simulink model "Quadcopter_V6"  (R2024b)
settings: Solver=FixedStepAuto  StartTime=0.0  StopTime=72  FixedStep=0.01  RelTol=1e-3  EnableMultiTasking=on
InitFcn:
  | QC_Params
values from neighbouring files (symbols this model uses):
  A_drag = [Ax 0  0 ... (first row only)    [QC_Params.m]
  b = 1.140e-7    (= 1.14e-07)    [QC_Params.m]
  g = 9.81    [QC_Params.m]
  grav = [0; 0; g]    [QC_Params.m]
  Ixx = 4.856e-3    (= 0.004856)    [QC_Params.m]
  Iyy = 4.856e-3    (= 0.004856)    [QC_Params.m]
  Izz = 8.801e-3    (= 0.008801)    [QC_Params.m]
  k = 2.980e-6    (= 2.98e-06)    [QC_Params.m]
  l = 0.225    [QC_Params.m]
  m = 0.468    [QC_Params.m]
  Psi = 0    [QC_Params.m]
  traj_markers = zeros(N, 8)    [QC_Params.m]
libraries: slpidlib x6, sharedtransform x1, uavutilslib x1
settings Model: Creator=acer  LastModifiedBy=acer

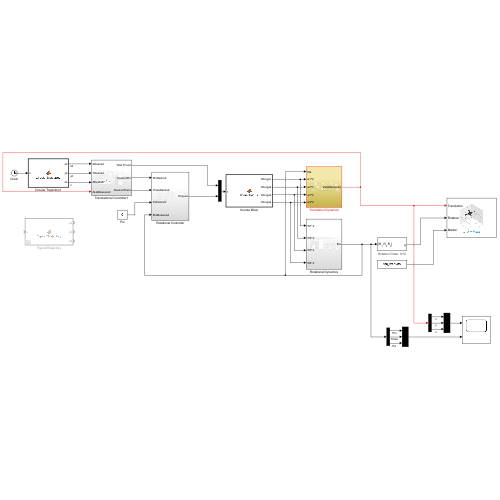
[thumbnail: Simulink's stored preview of the top-level diagram]
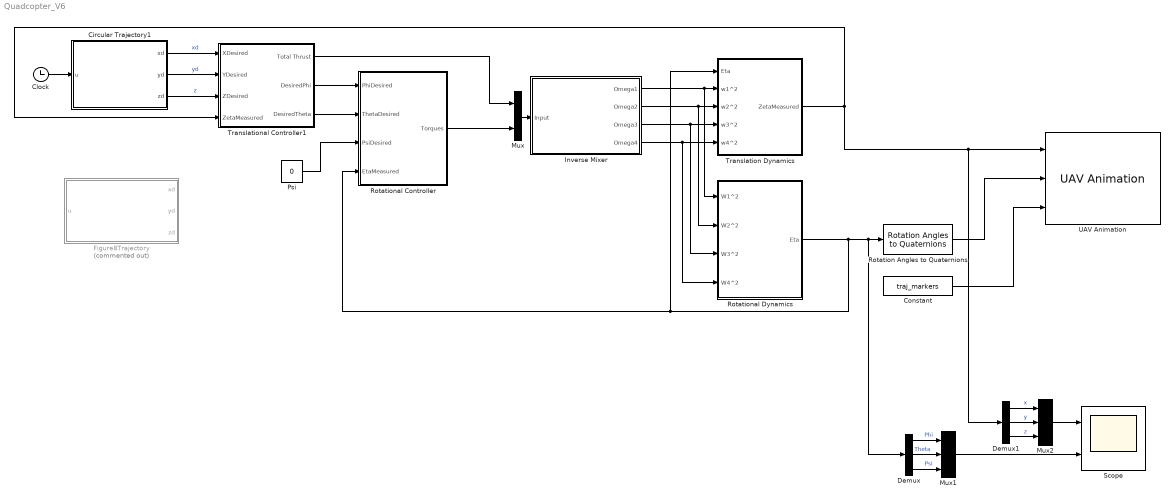
== system Quadcopter_V6 ==
  Circular Trajectory1 : MATLAB Function  TreatAsAtomicUnit=on
  Clock : Clock
  Constant : Constant  Value=traj_markers
  Demux : Demux  Outputs=3
  Demux1 : Demux  Outputs=3
  Figure8Trajectory : MATLAB Function  Commented=on  TreatAsAtomicUnit=on
  Inverse Mixer : MATLAB Function  TreatAsAtomicUnit=on
  Mux : Mux  Inputs=2
  Mux1 : Mux  Inputs=3
  Mux2 : Mux  Inputs=3
  Psi : Constant  Value=0
  Rotation Angles to Quaternions : sharedtransform/Rotation Angles to Quaternions  rotationOrder=XYZ  aMode=aMode
  Rotational Controller : Subsystem
  Rotational Dynamics : Subsystem
  Scope : Scope  NumInputPorts=2
  Translation Dynamics : Subsystem
  Translational Controller1 : Subsystem
  UAV Animation : uavutilslib/UAV Animation  NumUAV=1  DynamicUAVConfig=off  UAVType=Multirotor  UAVSize=2  UAVColor=[1 0 0]  UAVTrajectoryAlpha=1  InertialZDirection=Up  RotationFormat=Quaternion  DrawMarkers=on  SampleTime=-1
  wires:
  Inverse Mixer/1(Omega1) -> Rotational Dynamics/1(W1^2), Translation Dynamics/2(w1^2)
  Inverse Mixer/2(Omega2) -> Rotational Dynamics/2(W2^2), Translation Dynamics/3(w2^2)
  Inverse Mixer/3(Omega3) -> Rotational Dynamics/3(W3^2), Translation Dynamics/4(w3^2)
  Rotational Dynamics/1(Eta) -> Demux/1, Rotation Angles to Quaternions/1, Rotational Controller/4(EtaMeasured), Translation Dynamics/1(Eta)
  Mux/1 -> Inverse Mixer/1(Input)
  Inverse Mixer/4(Omega4) -> Rotational Dynamics/4(W4^2), Translation Dynamics/5(w4^2)
  Rotational Controller/1(Torques) -> Mux/2
  Translational Controller1/1(Total Thrust) -> Mux/1
  Translational Controller1/2(DesiredPhi) -> Rotational Controller/1(PhiDesired)
  Translational Controller1/3(DesiredTheta) -> Rotational Controller/2(ThetaDesired)
  Psi/1 -> Rotational Controller/3(PsiDesired)
  Constant/1 -> UAV Animation/3
  Circular Trajectory1/3(zd) -> Translational Controller1/3(ZDesired)  "z"
  Circular Trajectory1/1(xd) -> Translational Controller1/1(XDesired)  "xd"
  Circular Trajectory1/2(yd) -> Translational Controller1/2(YDesired)  "yd"
  Translation Dynamics/1(ZetaMeasured) -> Translational Controller1/4(ZetaMeasured), Demux1/1, UAV Animation/1
  Clock/1 -> Circular Trajectory1/1(u)
  Rotation Angles to Quaternions/1 -> UAV Animation/2
  Mux1/1 -> Scope/2
  Demux/2 -> Mux1/2  "Theta"
  Demux/1 -> Mux1/1  "Phi"
  Demux/3 -> Mux1/3  "Psi"
  Demux1/1 -> Mux2/1  "x"
  Demux1/2 -> Mux2/2  "y"
  Demux1/3 -> Mux2/3  "z"
  Mux2/1 -> Scope/1

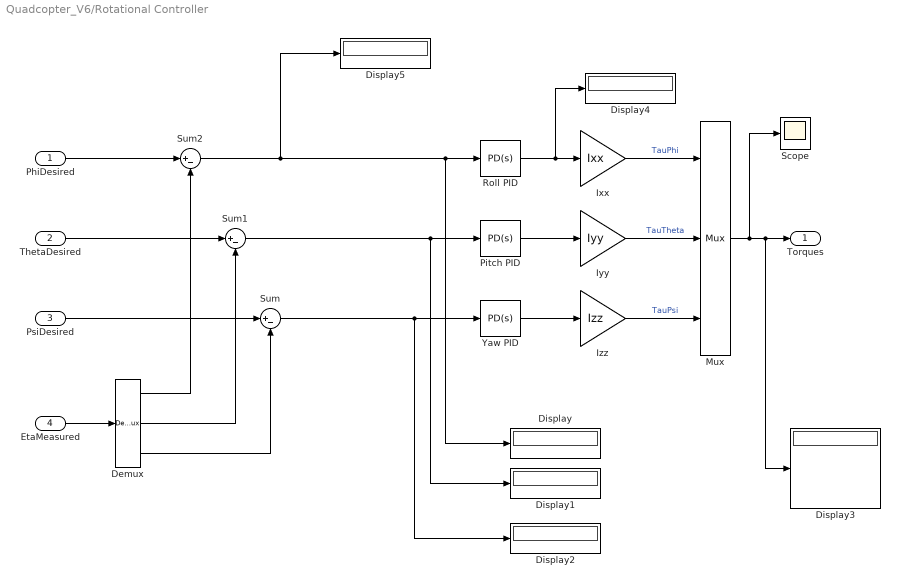
== system Quadcopter_V6/Rotational Controller ==
  PhiDesired : Inport
  ThetaDesired : Inport  Port=2
  PsiDesired : Inport  Port=3
  EtaMeasured : Inport  Port=4
  Demux : Demux  Outputs=3
  Display{,1..5} (6 alike) : Display
  Ixx : Gain  Gain=Ixx
  Iyy : Gain  Gain=Iyy
  Izz : Gain  Gain=Izz
  Mux : Mux  Inputs=3
  Pitch PID : slpidlib/PID Controller  Controller=PD  Form=Parallel  TimeDomain=Continuous-time  UseExternalTs=off  SampleTime=-1  IntegratorMethod=Forward Euler  FilterMethod=Forward Euler  ControllerParametersSource=internal  P=0.2  I=1.75  UseKiTs=off  D=10  UseExternalDerivativeSource=off  N=100  UseFilter=on  TunerSelectOption=Transfer Function Based (PID Tuner App)  InitialConditionSource=internal  InitialConditionForIntegrator=0  InitialConditionForFilter=0  DifferentiatorICPrevScaledInput=0  ExternalReset=none  TrackingMode=off  Kt=1  LimitOutput=off  SatLimitsSource=internal  UpperSaturationLimit=0.5  LowerSaturationLimit=-0.5  LinearizeAsGain=on  AntiWindupMode=none  Kb=1  LimitIntegrator=off  UpperIntegratorSaturationLimit=inf  LowerIntegratorSaturationLimit=-inf  POutMin=[]  POutMax=[]  IOutMin=[]  IOutMax=[]  DOutMin=[]  DOutMax=[]  NOutMin=[]  NOutMax=[]  SumOutMin=[]  SumOutMax=[]  SaturationOutMin=[]  SaturationOutMax=[]  PParamMin=[]  PParamMax=[]  IParamMin=[]  IParamMax=[]  DParamMin=[]  DParamMax=[]  NParamMin=[]  NParamMax=[]  KbParamMin=[]  KbParamMax=[]  KtParamMin=[]  KtParamMax=[]  KbOutMin=[]  KbOutMax=[]  KtOutMin=[]  KtOutMax=[]  IntegratorOutMin=[]  IntegratorOutMax=[]  FilterOutMin=[]  FilterOutMax=[]  SumI1OutMin=[]  SumI1OutMax=[]  SumI2OutMin=[]  SumI2OutMax=[]  SumI3OutMin=[]  SumI3OutMax=[]  SumI4OutMin=[]  SumI4OutMax=[]  SumDOutMin=[]  SumDOutMax=[]  DifferentiatorOutMin=[]  DifferentiatorOutMax=[]  FilterDiffOutCoefMin=[]  FilterDiffOutCoefMax=[]  ReciprocalOutMin=[]  ReciprocalOutMax=[]  SumDenOutMin=[]  SumDenOutMax=[]  SumNumOutMin=[]  SumNumOutMax=[]  DivideOutMin=[]  DivideOutMax=[]  UdiffTsProdOutMin=[]  UdiffTsProdOutMax=[]  NTsProdOutMin=[]  NTsProdOutMax=[]  UintegralTsProdOutMin=[]  UintegralTsProdOutMax=[]  UngainTsProdOutMin=[]  UngainTsProdOutMax=[]  ClampingZeroOutDataTypeStr=Inherit: Inherit via back propagation  ClampingZeroOutMin=[]  ClampingZeroOutMax=[]  FilterDenConstantOutDataTypeStr=Inherit: Inherit via back propagation  FilterDenConstantOutMin=[]  FilterDenConstantOutMax=[]  PCopyOutDataTypeStr=Inherit: Inherit via back propagation  PCopyOutMin=[]  PCopyOutMax=[]  NCopyOutDataTypeStr=Inherit: Inherit via back propagation  NCopyOutMin=[]  NCopyOutMax=[]  IntegratorContinuousStateAttributes=''  IntegratorStateMustResolveToSignalObject=off  IntegratorRTWStateStorageClass=Auto  FilterContinuousStateAttributes=''  FilterStateMustResolveToSignalObject=off  FilterRTWStateStorageClass=Auto  ParallelPVariant=InternalParameters  IdealPVariant=Disabled  IVariant=Disabled  DVariant=InternalParameters  IntegratorVariant=Disabled  SatVariant=Disabled  AWVariant=Disabled  PCopyVariant=Disabled  TRVariant=Disabled  FdbkBlocksVariant=Forward  IdealPFdbkVariant=Disabled  SatFdbkVariant=Disabled  DerivativeFilterVariant=ContFilter  NVariant=InternalParameters  NCopyVariant=Disabled  FilterICVariant=InternalICsFilter  IntegratorICVariant=Disabled  ExternalResetVariant=Disabled  TRSumVariant=Passthrough  SumFdbkVariant=Disabled  SumVariant=Sum_PD  TsampFilterVariant=InternalTs  TsampNgainVariant=Passthrough  TsampIntegralVariant=Disabled_SignalSpec  ExternalSaturationOutDataTypeStr=Inherit: Same as second input  DerivativeSourceVariant=ErrorSignal  PreIntVariant=InternalPreInt
  Roll PID : slpidlib/PID Controller  Controller=PD  Form=Parallel  TimeDomain=Continuous-time  UseExternalTs=off  SampleTime=-1  IntegratorMethod=Forward Euler  FilterMethod=Forward Euler  ControllerParametersSource=internal  P=0.2  I=0.15  UseKiTs=off  D=10  UseExternalDerivativeSource=off  N=100  UseFilter=on  TunerSelectOption=Transfer Function Based (PID Tuner App)  InitialConditionSource=internal  InitialConditionForIntegrator=0  InitialConditionForFilter=0  DifferentiatorICPrevScaledInput=0  ExternalReset=none  TrackingMode=off  Kt=1  LimitOutput=off  SatLimitsSource=internal  UpperSaturationLimit=0.5  LowerSaturationLimit=-0.5  LinearizeAsGain=on  AntiWindupMode=none  Kb=1  LimitIntegrator=off  UpperIntegratorSaturationLimit=inf  LowerIntegratorSaturationLimit=-inf  POutMin=[]  POutMax=[]  IOutMin=[]  IOutMax=[]  DOutMin=[]  DOutMax=[]  NOutMin=[]  NOutMax=[]  SumOutMin=[]  SumOutMax=[]  SaturationOutMin=[]  SaturationOutMax=[]  PParamMin=[]  PParamMax=[]  IParamMin=[]  IParamMax=[]  DParamMin=[]  DParamMax=[]  NParamMin=[]  NParamMax=[]  KbParamMin=[]  KbParamMax=[]  KtParamMin=[]  KtParamMax=[]  KbOutMin=[]  KbOutMax=[]  KtOutMin=[]  KtOutMax=[]  IntegratorOutMin=[]  IntegratorOutMax=[]  FilterOutMin=[]  FilterOutMax=[]  SumI1OutMin=[]  SumI1OutMax=[]  SumI2OutMin=[]  SumI2OutMax=[]  SumI3OutMin=[]  SumI3OutMax=[]  SumI4OutMin=[]  SumI4OutMax=[]  SumDOutMin=[]  SumDOutMax=[]  DifferentiatorOutMin=[]  DifferentiatorOutMax=[]  FilterDiffOutCoefMin=[]  FilterDiffOutCoefMax=[]  ReciprocalOutMin=[]  ReciprocalOutMax=[]  SumDenOutMin=[]  SumDenOutMax=[]  SumNumOutMin=[]  SumNumOutMax=[]  DivideOutMin=[]  DivideOutMax=[]  UdiffTsProdOutMin=[]  UdiffTsProdOutMax=[]  NTsProdOutMin=[]  NTsProdOutMax=[]  UintegralTsProdOutMin=[]  UintegralTsProdOutMax=[]  UngainTsProdOutMin=[]  UngainTsProdOutMax=[]  ClampingZeroOutDataTypeStr=Inherit: Inherit via back propagation  ClampingZeroOutMin=[]  ClampingZeroOutMax=[]  FilterDenConstantOutDataTypeStr=Inherit: Inherit via back propagation  FilterDenConstantOutMin=[]  FilterDenConstantOutMax=[]  PCopyOutDataTypeStr=Inherit: Inherit via back propagation  PCopyOutMin=[]  PCopyOutMax=[]  NCopyOutDataTypeStr=Inherit: Inherit via back propagation  NCopyOutMin=[]  NCopyOutMax=[]  IntegratorContinuousStateAttributes=''  IntegratorStateMustResolveToSignalObject=off  IntegratorRTWStateStorageClass=Auto  FilterContinuousStateAttributes=''  FilterStateMustResolveToSignalObject=off  FilterRTWStateStorageClass=Auto  ParallelPVariant=InternalParameters  IdealPVariant=Disabled  IVariant=Disabled  DVariant=InternalParameters  IntegratorVariant=Disabled  SatVariant=Disabled  AWVariant=Disabled  PCopyVariant=Disabled  TRVariant=Disabled  FdbkBlocksVariant=Forward  IdealPFdbkVariant=Disabled  SatFdbkVariant=Disabled  DerivativeFilterVariant=ContFilter  NVariant=InternalParameters  NCopyVariant=Disabled  FilterICVariant=InternalICsFilter  IntegratorICVariant=Disabled  ExternalResetVariant=Disabled  TRSumVariant=Passthrough  SumFdbkVariant=Disabled  SumVariant=Sum_PD  TsampFilterVariant=InternalTs  TsampNgainVariant=Passthrough  TsampIntegralVariant=Disabled_SignalSpec  ExternalSaturationOutDataTypeStr=Inherit: Same as second input  DerivativeSourceVariant=ErrorSignal  PreIntVariant=InternalPreInt
  Scope : Scope
  Sum : Sum  Inputs=|+-
  Sum1 : Sum  Inputs=|+-
  Sum2 : Sum  Inputs=|+-
  Yaw PID : slpidlib/PID Controller  Controller=PD  Form=Parallel  TimeDomain=Continuous-time  UseExternalTs=off  SampleTime=-1  IntegratorMethod=Forward Euler  FilterMethod=Forward Euler  ControllerParametersSource=internal  P=0.2  I=1  UseKiTs=off  D=10  UseExternalDerivativeSource=off  N=100  UseFilter=on  TunerSelectOption=Transfer Function Based (PID Tuner App)  InitialConditionSource=internal  InitialConditionForIntegrator=0  InitialConditionForFilter=0  DifferentiatorICPrevScaledInput=0  ExternalReset=none  TrackingMode=off  Kt=1  LimitOutput=off  SatLimitsSource=internal  UpperSaturationLimit=2*pi  LowerSaturationLimit=-2*pi  LinearizeAsGain=on  AntiWindupMode=none  Kb=1  LimitIntegrator=off  UpperIntegratorSaturationLimit=inf  LowerIntegratorSaturationLimit=-inf  POutMin=[]  POutMax=[]  IOutMin=[]  IOutMax=[]  DOutMin=[]  DOutMax=[]  NOutMin=[]  NOutMax=[]  SumOutMin=[]  SumOutMax=[]  SaturationOutMin=[]  SaturationOutMax=[]  PParamMin=[]  PParamMax=[]  IParamMin=[]  IParamMax=[]  DParamMin=[]  DParamMax=[]  NParamMin=[]  NParamMax=[]  KbParamMin=[]  KbParamMax=[]  KtParamMin=[]  KtParamMax=[]  KbOutMin=[]  KbOutMax=[]  KtOutMin=[]  KtOutMax=[]  IntegratorOutMin=[]  IntegratorOutMax=[]  FilterOutMin=[]  FilterOutMax=[]  SumI1OutMin=[]  SumI1OutMax=[]  SumI2OutMin=[]  SumI2OutMax=[]  SumI3OutMin=[]  SumI3OutMax=[]  SumI4OutMin=[]  SumI4OutMax=[]  SumDOutMin=[]  SumDOutMax=[]  DifferentiatorOutMin=[]  DifferentiatorOutMax=[]  FilterDiffOutCoefMin=[]  FilterDiffOutCoefMax=[]  ReciprocalOutMin=[]  ReciprocalOutMax=[]  SumDenOutMin=[]  SumDenOutMax=[]  SumNumOutMin=[]  SumNumOutMax=[]  DivideOutMin=[]  DivideOutMax=[]  UdiffTsProdOutMin=[]  UdiffTsProdOutMax=[]  NTsProdOutMin=[]  NTsProdOutMax=[]  UintegralTsProdOutMin=[]  UintegralTsProdOutMax=[]  UngainTsProdOutMin=[]  UngainTsProdOutMax=[]  ClampingZeroOutDataTypeStr=Inherit: Inherit via back propagation  ClampingZeroOutMin=[]  ClampingZeroOutMax=[]  FilterDenConstantOutDataTypeStr=Inherit: Inherit via back propagation  FilterDenConstantOutMin=[]  FilterDenConstantOutMax=[]  PCopyOutDataTypeStr=Inherit: Inherit via back propagation  PCopyOutMin=[]  PCopyOutMax=[]  NCopyOutDataTypeStr=Inherit: Inherit via back propagation  NCopyOutMin=[]  NCopyOutMax=[]  IntegratorContinuousStateAttributes=''  IntegratorStateMustResolveToSignalObject=off  IntegratorRTWStateStorageClass=Auto  FilterContinuousStateAttributes=''  FilterStateMustResolveToSignalObject=off  FilterRTWStateStorageClass=Auto  ParallelPVariant=InternalParameters  IdealPVariant=Disabled  IVariant=Disabled  DVariant=InternalParameters  IntegratorVariant=Disabled  SatVariant=Disabled  AWVariant=Disabled  PCopyVariant=Disabled  TRVariant=Disabled  FdbkBlocksVariant=Forward  IdealPFdbkVariant=Disabled  SatFdbkVariant=Disabled  DerivativeFilterVariant=ContFilter  NVariant=InternalParameters  NCopyVariant=Disabled  FilterICVariant=InternalICsFilter  IntegratorICVariant=Disabled  ExternalResetVariant=Disabled  TRSumVariant=Passthrough  SumFdbkVariant=Disabled  SumVariant=Sum_PD  TsampFilterVariant=InternalTs  TsampNgainVariant=Passthrough  TsampIntegralVariant=Disabled_SignalSpec  ExternalSaturationOutDataTypeStr=Inherit: Same as second input  DerivativeSourceVariant=ErrorSignal  PreIntVariant=InternalPreInt
  Torques : Outport
  wires:
  EtaMeasured/1 -> Demux/1
  PsiDesired/1 -> Sum/1
  ThetaDesired/1 -> Sum1/1
  PhiDesired/1 -> Sum2/1
  Sum2/1 -> Display5/1, Display/1, Roll PID/1
  Sum1/1 -> Display1/1, Pitch PID/1
  Sum/1 -> Display2/1, Yaw PID/1
  Roll PID/1 -> Display4/1, Ixx/1
  Pitch PID/1 -> Iyy/1
  Yaw PID/1 -> Izz/1
  Izz/1 -> Mux/3  "TauPsi"
  Iyy/1 -> Mux/2  "TauTheta"
  Ixx/1 -> Mux/1  "TauPhi"
  Mux/1 -> Scope/1, Display3/1, Torques/1
  Demux/1 -> Sum2/2
  Demux/2 -> Sum1/2
  Demux/3 -> Sum/2

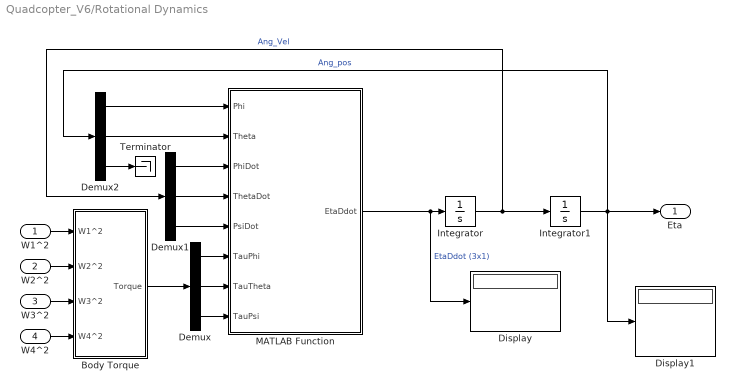
== system Quadcopter_V6/Rotational Dynamics ==
  W1^2 : Inport
  W2^2 : Inport  Port=2
  W3^2 : Inport  Port=3
  W4^2 : Inport  Port=4
  Body Torque : Subsystem
  Demux : Demux  Outputs=3
  Demux1 : Demux  Outputs=3
  Demux2 : Demux  Outputs=3
  Display : Display
  Display1 : Display
  Integrator : Integrator  InitialCondition=[0;0;0]  IgnoreLimit=on
  Integrator1 : Integrator  InitialCondition=[0;0;0]
  MATLAB Function : MATLAB Function  TreatAsAtomicUnit=on
  Terminator : Terminator
  Eta : Outport
  wires:
  W1^2/1 -> Body Torque/1(W1^2)
  W2^2/1 -> Body Torque/2(W2^2)
  W3^2/1 -> Body Torque/3(W3^2)
  W4^2/1 -> Body Torque/4(W4^2)
  Body Torque/1(Torque) -> Demux/1
  Integrator/1 -> Integrator1/1, Demux1/1  "Ang_Vel"
  Integrator1/1 -> Display1/1, Demux2/1, Eta/1  "Ang_pos"
  Demux2/1 -> MATLAB Function/1(Phi)
  Demux2/3 -> Terminator/1
  Demux/1 -> MATLAB Function/6(TauPhi)
  Demux/2 -> MATLAB Function/7(TauTheta)
  Demux/3 -> MATLAB Function/8(TauPsi)
  Demux1/2 -> MATLAB Function/4(ThetaDot)
  Demux1/1 -> MATLAB Function/3(PhiDot)
  Demux2/2 -> MATLAB Function/2(Theta)
  Demux1/3 -> MATLAB Function/5(PsiDot)
  MATLAB Function/1(EtaDdot) -> Display/1, Integrator/1  "EtaDdot (3x1)"

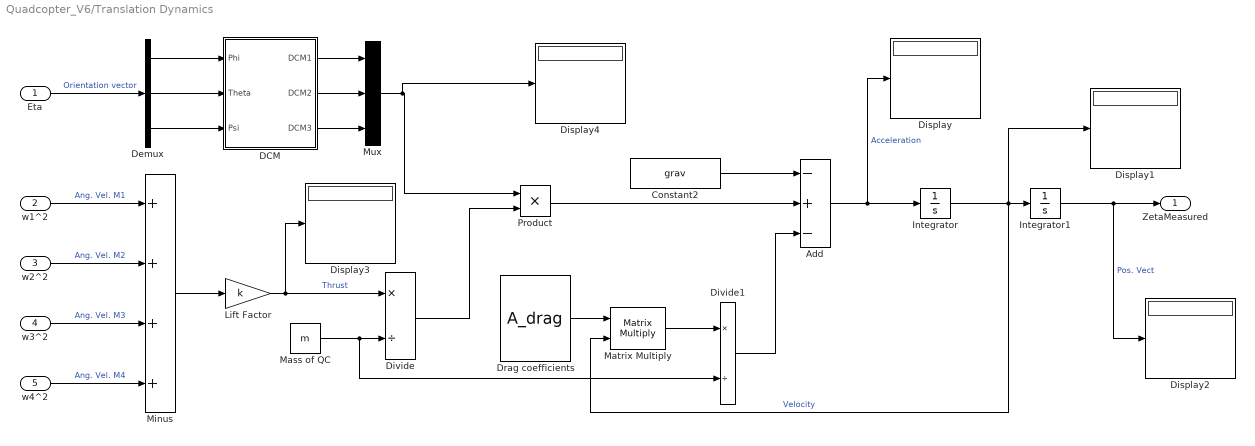
== system Quadcopter_V6/Translation Dynamics ==
  Eta : Inport
  w1^2 : Inport  Port=2
  w2^2 : Inport  Port=3
  w3^2 : Inport  Port=4
  w4^2 : Inport  Port=5
  Add : Sum  Inputs=-+-
  Constant2 : Constant  Value=grav
  "DCM " : MATLAB Function  TreatAsAtomicUnit=on
  Demux : Demux  Outputs=3
  Display{,1..4} (5 alike) : Display
  Divide : Product  Inputs=*/
  Divide1 : Product  Inputs=*/
  Drag coefficients : Constant  Value=A_drag
  Integrator : Integrator  InitialCondition=[0;0;0]
  Integrator1 : Integrator  InitialCondition=[0;0;0]
  Lift Factor : Gain  Gain=k
  Mass of QC : Constant  Value=m
  Matrix Multiply : Product  Multiplication=Matrix(*)
  Minus : Sum  Inputs=++++
  Mux : Mux  Inputs=3
  Product : Product
  ZetaMeasured : Outport
  wires:
  w1^2/1 -> Minus/1  "Ang. Vel. M1"
  w2^2/1 -> Minus/2  "Ang. Vel. M2"
  w3^2/1 -> Minus/3  "Ang. Vel. M3"
  w4^2/1 -> Minus/4  "Ang. Vel. M4"
  Minus/1 -> Lift Factor/1
  Eta/1 -> Demux/1  "Orientation vector"
  Demux/3 -> "DCM "/3(Psi)
  Demux/2 -> "DCM "/2(Theta)
  Demux/1 -> "DCM "/1(Phi)
  Lift Factor/1 -> Display3/1, Divide/1  "Thrust"
  Mass of QC/1 -> Divide1/2, Divide/2
  Divide/1 -> Product/2
  Drag coefficients/1 -> Matrix Multiply/1
  Matrix Multiply/1 -> Divide1/1
  Constant2/1 -> Add/1
  Product/1 -> Add/2
  Divide1/1 -> Add/3
  Add/1 -> Display/1, Integrator/1  "Acceleration"
  Integrator/1 -> Display1/1, Matrix Multiply/2, Integrator1/1  "Velocity"
  Integrator1/1 -> Display2/1, ZetaMeasured/1  "Pos. Vect"
  Mux/1 -> Display4/1, Product/1
  "DCM "/1(DCM1) -> Mux/1
  "DCM "/2(DCM2) -> Mux/2
  "DCM "/3(DCM3) -> Mux/3

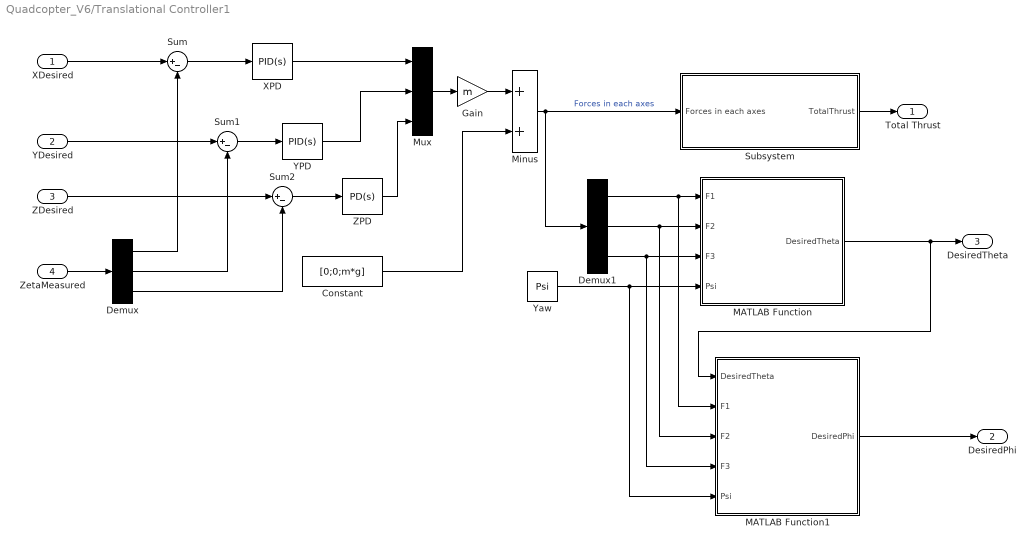
== system Quadcopter_V6/Translational Controller1 ==
  XDesired : Inport
  YDesired : Inport  Port=2
  ZDesired : Inport  Port=3
  ZetaMeasured : Inport  Port=4
  Constant : Constant  Value=[0;0;m*g]
  Demux : Demux  Outputs=3
  Demux1 : Demux  Outputs=3
  Gain : Gain  Gain=m
  MATLAB Function : MATLAB Function  TreatAsAtomicUnit=on
  MATLAB Function1 : MATLAB Function  TreatAsAtomicUnit=on
  Minus : Sum
  Mux : Mux  Inputs=3
  Subsystem : Subsystem
  Sum : Sum  Inputs=|+-
  Sum1 : Sum  Inputs=|+-
  Sum2 : Sum  Inputs=|+-
  XPD : slpidlib/PID Controller  Controller=PID  Form=Parallel  TimeDomain=Continuous-time  UseExternalTs=off  SampleTime=-1  IntegratorMethod=Forward Euler  FilterMethod=Forward Euler  ControllerParametersSource=internal  P=10  I=1  UseKiTs=off  D=20  UseExternalDerivativeSource=off  N=100  UseFilter=on  TunerSelectOption=Transfer Function Based (PID Tuner App)  InitialConditionSource=internal  InitialConditionForIntegrator=0  InitialConditionForFilter=0  DifferentiatorICPrevScaledInput=0  ExternalReset=none  TrackingMode=off  Kt=1  LimitOutput=off  SatLimitsSource=internal  UpperSaturationLimit=inf  LowerSaturationLimit=-inf  LinearizeAsGain=on  AntiWindupMode=none  Kb=1  LimitIntegrator=off  UpperIntegratorSaturationLimit=inf  LowerIntegratorSaturationLimit=-inf  POutMin=[]  POutMax=[]  IOutMin=[]  IOutMax=[]  DOutMin=[]  DOutMax=[]  NOutMin=[]  NOutMax=[]  SumOutMin=[]  SumOutMax=[]  SaturationOutMin=[]  SaturationOutMax=[]  PParamMin=[]  PParamMax=[]  IParamMin=[]  IParamMax=[]  DParamMin=[]  DParamMax=[]  NParamMin=[]  NParamMax=[]  KbParamMin=[]  KbParamMax=[]  KtParamMin=[]  KtParamMax=[]  KbOutMin=[]  KbOutMax=[]  KtOutMin=[]  KtOutMax=[]  IntegratorOutMin=[]  IntegratorOutMax=[]  FilterOutMin=[]  FilterOutMax=[]  SumI1OutMin=[]  SumI1OutMax=[]  SumI2OutMin=[]  SumI2OutMax=[]  SumI3OutMin=[]  SumI3OutMax=[]  SumI4OutMin=[]  SumI4OutMax=[]  SumDOutMin=[]  SumDOutMax=[]  DifferentiatorOutMin=[]  DifferentiatorOutMax=[]  FilterDiffOutCoefMin=[]  FilterDiffOutCoefMax=[]  ReciprocalOutMin=[]  ReciprocalOutMax=[]  SumDenOutMin=[]  SumDenOutMax=[]  SumNumOutMin=[]  SumNumOutMax=[]  DivideOutMin=[]  DivideOutMax=[]  UdiffTsProdOutMin=[]  UdiffTsProdOutMax=[]  NTsProdOutMin=[]  NTsProdOutMax=[]  UintegralTsProdOutMin=[]  UintegralTsProdOutMax=[]  UngainTsProdOutMin=[]  UngainTsProdOutMax=[]  ClampingZeroOutDataTypeStr=Inherit: Inherit via back propagation  ClampingZeroOutMin=[]  ClampingZeroOutMax=[]  FilterDenConstantOutDataTypeStr=Inherit: Inherit via back propagation  FilterDenConstantOutMin=[]  FilterDenConstantOutMax=[]  PCopyOutDataTypeStr=Inherit: Inherit via back propagation  PCopyOutMin=[]  PCopyOutMax=[]  NCopyOutDataTypeStr=Inherit: Inherit via back propagation  NCopyOutMin=[]  NCopyOutMax=[]  IntegratorContinuousStateAttributes=''  IntegratorStateMustResolveToSignalObject=off  IntegratorRTWStateStorageClass=Auto  FilterContinuousStateAttributes=''  FilterStateMustResolveToSignalObject=off  FilterRTWStateStorageClass=Auto  ParallelPVariant=InternalParameters  IdealPVariant=Disabled  IVariant=InternalParameters  DVariant=InternalParameters  IntegratorVariant=Continuous  SatVariant=Disabled  AWVariant=Passthrough  PCopyVariant=Disabled  TRVariant=Disabled  FdbkBlocksVariant=Forward  IdealPFdbkVariant=Disabled  SatFdbkVariant=Disabled  DerivativeFilterVariant=ContFilter  NVariant=InternalParameters  NCopyVariant=Disabled  FilterICVariant=InternalICsFilter  IntegratorICVariant=InternalICs  ExternalResetVariant=Disabled  TRSumVariant=Passthrough  SumFdbkVariant=Disabled  SumVariant=Sum_PID  TsampFilterVariant=InternalTs  TsampNgainVariant=Passthrough  TsampIntegralVariant=Disabled_SignalSpec  ExternalSaturationOutDataTypeStr=Inherit: Same as second input  DerivativeSourceVariant=ErrorSignal  PreIntVariant=InternalPreInt
  YPD : slpidlib/PID Controller  Controller=PID  Form=Parallel  TimeDomain=Continuous-time  UseExternalTs=off  SampleTime=-1  IntegratorMethod=Forward Euler  FilterMethod=Forward Euler  ControllerParametersSource=internal  P=5  I=2  UseKiTs=off  D=4  UseExternalDerivativeSource=off  N=100  UseFilter=on  TunerSelectOption=Transfer Function Based (PID Tuner App)  InitialConditionSource=internal  InitialConditionForIntegrator=0  InitialConditionForFilter=0  DifferentiatorICPrevScaledInput=0  ExternalReset=none  TrackingMode=off  Kt=1  LimitOutput=off  SatLimitsSource=internal  UpperSaturationLimit=inf  LowerSaturationLimit=-inf  LinearizeAsGain=on  AntiWindupMode=none  Kb=1  LimitIntegrator=off  UpperIntegratorSaturationLimit=inf  LowerIntegratorSaturationLimit=-inf  POutMin=[]  POutMax=[]  IOutMin=[]  IOutMax=[]  DOutMin=[]  DOutMax=[]  NOutMin=[]  NOutMax=[]  SumOutMin=[]  SumOutMax=[]  SaturationOutMin=[]  SaturationOutMax=[]  PParamMin=[]  PParamMax=[]  IParamMin=[]  IParamMax=[]  DParamMin=[]  DParamMax=[]  NParamMin=[]  NParamMax=[]  KbParamMin=[]  KbParamMax=[]  KtParamMin=[]  KtParamMax=[]  KbOutMin=[]  KbOutMax=[]  KtOutMin=[]  KtOutMax=[]  IntegratorOutMin=[]  IntegratorOutMax=[]  FilterOutMin=[]  FilterOutMax=[]  SumI1OutMin=[]  SumI1OutMax=[]  SumI2OutMin=[]  SumI2OutMax=[]  SumI3OutMin=[]  SumI3OutMax=[]  SumI4OutMin=[]  SumI4OutMax=[]  SumDOutMin=[]  SumDOutMax=[]  DifferentiatorOutMin=[]  DifferentiatorOutMax=[]  FilterDiffOutCoefMin=[]  FilterDiffOutCoefMax=[]  ReciprocalOutMin=[]  ReciprocalOutMax=[]  SumDenOutMin=[]  SumDenOutMax=[]  SumNumOutMin=[]  SumNumOutMax=[]  DivideOutMin=[]  DivideOutMax=[]  UdiffTsProdOutMin=[]  UdiffTsProdOutMax=[]  NTsProdOutMin=[]  NTsProdOutMax=[]  UintegralTsProdOutMin=[]  UintegralTsProdOutMax=[]  UngainTsProdOutMin=[]  UngainTsProdOutMax=[]  ClampingZeroOutDataTypeStr=Inherit: Inherit via back propagation  ClampingZeroOutMin=[]  ClampingZeroOutMax=[]  FilterDenConstantOutDataTypeStr=Inherit: Inherit via back propagation  FilterDenConstantOutMin=[]  FilterDenConstantOutMax=[]  PCopyOutDataTypeStr=Inherit: Inherit via back propagation  PCopyOutMin=[]  PCopyOutMax=[]  NCopyOutDataTypeStr=Inherit: Inherit via back propagation  NCopyOutMin=[]  NCopyOutMax=[]  IntegratorContinuousStateAttributes=''  IntegratorStateMustResolveToSignalObject=off  IntegratorRTWStateStorageClass=Auto  FilterContinuousStateAttributes=''  FilterStateMustResolveToSignalObject=off  FilterRTWStateStorageClass=Auto  ParallelPVariant=InternalParameters  IdealPVariant=Disabled  IVariant=InternalParameters  DVariant=InternalParameters  IntegratorVariant=Continuous  SatVariant=Disabled  AWVariant=Passthrough  PCopyVariant=Disabled  TRVariant=Disabled  FdbkBlocksVariant=Forward  IdealPFdbkVariant=Disabled  SatFdbkVariant=Disabled  DerivativeFilterVariant=ContFilter  NVariant=InternalParameters  NCopyVariant=Disabled  FilterICVariant=InternalICsFilter  IntegratorICVariant=InternalICs  ExternalResetVariant=Disabled  TRSumVariant=Passthrough  SumFdbkVariant=Disabled  SumVariant=Sum_PID  TsampFilterVariant=InternalTs  TsampNgainVariant=Passthrough  TsampIntegralVariant=Disabled_SignalSpec  ExternalSaturationOutDataTypeStr=Inherit: Same as second input  DerivativeSourceVariant=ErrorSignal  PreIntVariant=InternalPreInt
  Yaw : Constant  Value=Psi
  ZPD : slpidlib/PID Controller  Controller=PD  Form=Parallel  TimeDomain=Continuous-time  UseExternalTs=off  SampleTime=-1  IntegratorMethod=Forward Euler  FilterMethod=Forward Euler  ControllerParametersSource=internal  P=3.25  I=0.5  UseKiTs=off  D=2.5  UseExternalDerivativeSource=off  N=100  UseFilter=on  TunerSelectOption=Transfer Function Based (PID Tuner App)  InitialConditionSource=internal  InitialConditionForIntegrator=0  InitialConditionForFilter=0  DifferentiatorICPrevScaledInput=0  ExternalReset=none  TrackingMode=off  Kt=1  LimitOutput=off  SatLimitsSource=internal  UpperSaturationLimit=inf  LowerSaturationLimit=-inf  LinearizeAsGain=on  AntiWindupMode=none  Kb=1  LimitIntegrator=off  UpperIntegratorSaturationLimit=inf  LowerIntegratorSaturationLimit=-inf  POutMin=[]  POutMax=[]  IOutMin=[]  IOutMax=[]  DOutMin=[]  DOutMax=[]  NOutMin=[]  NOutMax=[]  SumOutMin=[]  SumOutMax=[]  SaturationOutMin=[]  SaturationOutMax=[]  PParamMin=[]  PParamMax=[]  IParamMin=[]  IParamMax=[]  DParamMin=[]  DParamMax=[]  NParamMin=[]  NParamMax=[]  KbParamMin=[]  KbParamMax=[]  KtParamMin=[]  KtParamMax=[]  KbOutMin=[]  KbOutMax=[]  KtOutMin=[]  KtOutMax=[]  IntegratorOutMin=[]  IntegratorOutMax=[]  FilterOutMin=[]  FilterOutMax=[]  SumI1OutMin=[]  SumI1OutMax=[]  SumI2OutMin=[]  SumI2OutMax=[]  SumI3OutMin=[]  SumI3OutMax=[]  SumI4OutMin=[]  SumI4OutMax=[]  SumDOutMin=[]  SumDOutMax=[]  DifferentiatorOutMin=[]  DifferentiatorOutMax=[]  FilterDiffOutCoefMin=[]  FilterDiffOutCoefMax=[]  ReciprocalOutMin=[]  ReciprocalOutMax=[]  SumDenOutMin=[]  SumDenOutMax=[]  SumNumOutMin=[]  SumNumOutMax=[]  DivideOutMin=[]  DivideOutMax=[]  UdiffTsProdOutMin=[]  UdiffTsProdOutMax=[]  NTsProdOutMin=[]  NTsProdOutMax=[]  UintegralTsProdOutMin=[]  UintegralTsProdOutMax=[]  UngainTsProdOutMin=[]  UngainTsProdOutMax=[]  ClampingZeroOutDataTypeStr=Inherit: Inherit via back propagation  ClampingZeroOutMin=[]  ClampingZeroOutMax=[]  FilterDenConstantOutDataTypeStr=Inherit: Inherit via back propagation  FilterDenConstantOutMin=[]  FilterDenConstantOutMax=[]  PCopyOutDataTypeStr=Inherit: Inherit via back propagation  PCopyOutMin=[]  PCopyOutMax=[]  NCopyOutDataTypeStr=Inherit: Inherit via back propagation  NCopyOutMin=[]  NCopyOutMax=[]  IntegratorContinuousStateAttributes=''  IntegratorStateMustResolveToSignalObject=off  IntegratorRTWStateStorageClass=Auto  FilterContinuousStateAttributes=''  FilterStateMustResolveToSignalObject=off  FilterRTWStateStorageClass=Auto  ParallelPVariant=InternalParameters  IdealPVariant=Disabled  IVariant=Disabled  DVariant=InternalParameters  IntegratorVariant=Disabled  SatVariant=Disabled  AWVariant=Disabled  PCopyVariant=Disabled  TRVariant=Disabled  FdbkBlocksVariant=Forward  IdealPFdbkVariant=Disabled  SatFdbkVariant=Disabled  DerivativeFilterVariant=ContFilter  NVariant=InternalParameters  NCopyVariant=Disabled  FilterICVariant=InternalICsFilter  IntegratorICVariant=Disabled  ExternalResetVariant=Disabled  TRSumVariant=Passthrough  SumFdbkVariant=Disabled  SumVariant=Sum_PD  TsampFilterVariant=InternalTs  TsampNgainVariant=Passthrough  TsampIntegralVariant=Disabled_SignalSpec  ExternalSaturationOutDataTypeStr=Inherit: Same as second input  DerivativeSourceVariant=ErrorSignal  PreIntVariant=InternalPreInt
  Total Thrust : Outport
  DesiredPhi : Outport  Port=2
  DesiredTheta : Outport  Port=3
  wires:
  ZetaMeasured/1 -> Demux/1
  XDesired/1 -> Sum/1
  Demux/1 -> Sum/2
  YDesired/1 -> Sum1/1
  Demux/2 -> Sum1/2
  Demux/3 -> Sum2/2
  ZDesired/1 -> Sum2/1
  Sum/1 -> XPD/1
  Sum1/1 -> YPD/1
  Sum2/1 -> ZPD/1
  Constant/1 -> Minus/2
  ZPD/1 -> Mux/3
  YPD/1 -> Mux/2
  XPD/1 -> Mux/1
  Mux/1 -> Gain/1
  Gain/1 -> Minus/1
  Minus/1 -> Subsystem/1(Forces in each axes), Demux1/1  "Forces in each axes"
  Subsystem/1(TotalThrust) -> Total Thrust/1
  Demux1/1 -> MATLAB Function1/2(F1), MATLAB Function/1(F1)
  Demux1/2 -> MATLAB Function1/3(F2), MATLAB Function/2(F2)
  Demux1/3 -> MATLAB Function1/4(F3), MATLAB Function/3(F3)
  Yaw/1 -> MATLAB Function1/5(Psi), MATLAB Function/4(Psi)
  MATLAB Function/1(DesiredTheta) -> DesiredTheta/1, MATLAB Function1/1(DesiredTheta)
  MATLAB Function1/1(DesiredPhi) -> DesiredPhi/1

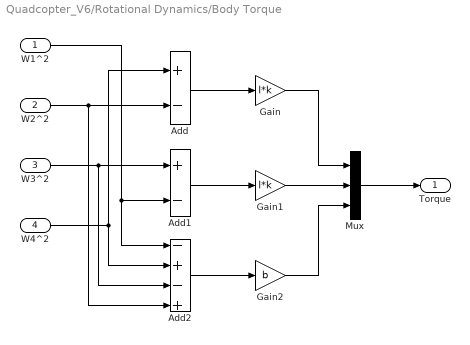
== system Quadcopter_V6/Rotational Dynamics/Body Torque ==
  W1^2 : Inport
  W2^2 : Inport  Port=2
  W3^2 : Inport  Port=3
  W4^2 : Inport  Port=4
  Add : Sum  Inputs=+-
  Add1 : Sum  Inputs=+-
  Add2 : Sum  Inputs=-+-+
  Gain : Gain  Gain=l*k
  Gain1 : Gain  Gain=l*k
  Gain2 : Gain  Gain=b
  Mux : Mux  Inputs=3
  Torque : Outport
  wires:
  Gain/1 -> Mux/1
  W1^2/1 -> Add1/2, Add2/1
  Add2/1 -> Gain2/1
  W4^2/1 -> Add2/2, Add/1
  W3^2/1 -> Add1/1, Add2/3
  W2^2/1 -> Add/2, Add2/4
  Add/1 -> Gain/1
  Add1/1 -> Gain1/1
  Gain1/1 -> Mux/2
  Gain2/1 -> Mux/3
  Mux/1 -> Torque/1

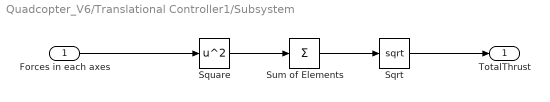
== system Quadcopter_V6/Translational Controller1/Subsystem ==
  Forces in each axes : Inport
  Sqrt : Sqrt
  Square : Math  Operator=square
  Sum of Elements : Sum  Inputs=+
  TotalThrust : Outport
  wires:
  Forces in each axes/1 -> Square/1
  Square/1 -> Sum of Elements/1
  Sum of Elements/1 -> Sqrt/1
  Sqrt/1 -> TotalThrust/1

== matlab function Quadcopter_V6/Translation Dynamics/DCM  ==
  data: Phi input; DCM1 output; Theta input; Psi input; DCM2 output; DCM3 output
function [DCM1, DCM2, DCM3] = Etta(Phi, Theta, Psi)

cp = cos(Phi);
sp = sin(Phi);
ct = cos(Theta);
st = sin(Theta);
cs = cos(Psi);
ss = sin(Psi);

DCM1 = cp*st*cs + sp*ss;
DCM2 = cp*st*ss - sp*cs;
DCM3 = cp*ct;
end

== matlab function Quadcopter_V6/Rotational Dynamics/MATLAB Function ==
  data: Phi input; EtaDdot output; Theta input; PhiDot input; ThetaDot input; PsiDot input; TauPhi input; TauTheta input; TauPsi input
function EtaDdot  = Quad(Phi, Theta, PhiDot, ThetaDot, PsiDot, TauPhi, TauTheta, TauPsi)
% Inertia constants (hardcoded for now — use Parameter scope later)
Ixx = 4.856e-3;
Iyy = 4.856e-3;
Izz = 8.801e-3;

% rest of code...


J = zeros(3,3); % Generalized mass matrix
%Formula for GMM, CCM
% Trig shorthand
%% Real Code
sp = sin(Phi);   cp = cos(Phi);
st = sin(Theta); ct = cos(Theta);
%%
%% Test Value
%sp = 0;   
%cp = 1;
%st = 0; 
%ct = 1;
%%


% Build J element by element
J = zeros(3,3);
J(1,1) = Ixx;
J(1,2) = 0;
J(1,3) = -Ixx*st;
J(2,1) = 0;
J(2,2) = Iyy*cp^2 + Izz*sp^2;
J(2,3) = (Iyy-Izz)*cp*sp*ct;
J(3,1) = -Ixx*st;
J(3,2) = (Iyy-Izz)*cp*sp*ct;
J(3,3) = Ixx*st^2 + Iyy*sp^2*ct^2 + Izz*cp^2*ct^2;

%Build C element
C = zeros(3, 3);            %Coriolis-centripetal matrix
%% Real Code
spcp   = sp*cp;             % sin(phi)*cos(phi)
sp2    = sp^2;              % sin^2(phi)
cp2    = cp^2;              % cos^2(phi)
ct2    = ct^2;              % cos^2(theta)
stct   = st*ct;             % sin(theta)*cos(theta)
%%
%% Test Value
%spcp   = 0;             % sin(phi)*cos(phi)
%sp2    = 0;              % sin^2(phi)
%cp2    = 1;              % cos^2(phi)
%ct2    = 1;              % cos^2(theta)
%stct   = 0;             % sin(theta)*cos(theta)
%%
%%
Iyz = Iyy - Izz;              % appears as (Iy-Iz)
Izy = Izz - Iyy;              % appears as (Iz-Iy) = -Iyz

% Build C element by element
C(1,1) = 0;

C(1,2) = Iyz*(ThetaDot*spcp + PsiDot*sp2*ct) + Izy*PsiDot*cp2*ct ...
       - Ixx*PsiDot*ct;

C(1,3) = Izy*PsiDot*spcp*ct2;

C(2,1) = Izy*(ThetaDot*spcp + PsiDot*sp*ct) + Iyz*PsiDot*cp2*ct ...
       + Ixx*PsiDot*ct;

C(2,2) = Izy*PhiDot*spcp;

C(2,3) = -Ixx*PsiDot*stct + Iyy*PsiDot*sp2*stct ...
       + Izz*PsiDot*cp2*stct;

C(3,1) = Iyz*PsiDot*ct2*spcp - Ixx*ThetaDot*ct;

C(3,2) = Izy*(ThetaDot*spcp*st + PhiDot*sp2*ct) + Iyz*PhiDot*cp2*ct ...
       + Ixx*PsiDot*stct - Iyy*PsiDot*sp2*stct - Izz*PsiDot*cp2*stct;

C(3,3) = Iyz*PhiDot*spcp*ct2 - Iyy*ThetaDot*sp2*stct ...
       - Izz*ThetaDot*cp2*stct + Ixx*ThetaDot*stct;

B = [TauPhi; TauTheta; TauPsi]; %Torque matrix
N = [PhiDot; ThetaDot; PsiDot];
EtaDdot = [inv(J)*(B-C*N)];

end

== matlab function Quadcopter_V6/Inverse Mixer ==
  data: Input input; Omega1 output; b parameter size=1; l parameter size=1; k parameter size=1; Omega2 output; Omega3 output; Omega4 output
function [Omega1, Omega2, Omega3, Omega4] = ThrustTorque(Input, b, l, k)

T        = Input(1);
TauPhi   = Input(2);
TauTheta = Input(3);
TauPsi   = Input(4);

T1 = T/(4*k);
TauP = TauPhi/(2*k*l);
TauT = TauTheta/(2*k*l);
TauS = TauPsi/(4*b);
Omega1 = T1 - TauT - TauS;
Omega2= T1 - TauP + TauS;
Omega3 = T1 + TauT - TauS;
Omega4 = T1 + TauP + TauS;
end
%% This function can be called inverse mixer, takes the torques and thrust
%% and gives the square of angular speed of each motor required to be operated at.

== matlab function Quadcopter_V6/Figure8Trajectory ==
  data: u input; xd output; yd output; zd output
function [xd, yd, zd] = Figure8Trajectory(u)
xd = 0;
yd = 0;
zd = 0;

% Phase 1: Climb from (0,0,0) to (0,0,10) in 10 seconds
if u < 10
    xd = 0;
    yd = 0;
    zd = u;
end


if u >= 10
    tau   = u - 10;
    omega = 2 * pi / 40;   % rad/s  —  period = 40 s
    R     = 6;              % m      —  lobe radius

    xd = R * sin(2*omega * tau);
    yd =  R * sin(omega * tau);
    zd = 10;
end

== matlab function Quadcopter_V6/Circular Trajectory1 ==
  data: u input; xd output; yd output; zd output
function [xd, yd, zd] = CircularTrajectory(u)

xd = 0;
yd = 0;
zd = 0;

% Climb from (0,0,0) to (0,0,10) in 10 seconds
if u < 10
    xd = 0;
    yd = 0;
    zd = u;
end

% Translate from (0,0,10) to (10,0,10) in 4 seconds
if u >= 10 && u < 14
    xd = 2.5 * (u - 10);
    yd = 0;
    zd = 10;
end

% Circular path of radius 10 at height 10
if u >= 14
    xd = 10 * cos(2*pi*(u - 14)/55);
    yd = 10 * sin(2*pi*(u - 14)/55);
    zd = 10;
end

== matlab function Quadcopter_V6/Translational Controller1/MATLAB Function ==
  data: F1 input; F2 input; F3 input; Psi input; DesiredTheta output
function DesiredTheta = ThetaCalculator(F1, F2, F3, Psi)

cs = cos(Psi);
ss = sin(Psi);
DesiredTheta = atan((F1*cs + F2*ss)/F3);

end

== matlab function Quadcopter_V6/Translational Controller1/MATLAB Function1 ==
  data: DesiredTheta input; F1 input; DesiredPhi output; F2 input; F3 input; Psi input
function DesiredPhi = PhiCalulator(DesiredTheta, F1, F2, F3, Psi)
cs = cos(Psi);
ss = sin(Psi);
ct = cos(DesiredTheta);
DesiredPhi  = atan((F1*ss - F2*cs)*ct/F3);
end
